simulink model "VelocityControl"  (R2018a)
settings: Solver=VariableStepAuto  StartTime=0.0  StopTime=10.0  RelTol=1e-3
values from neighbouring files (symbols this model uses):
  Dr = 30000    [BoatSim_config.m]    (also in WAM_V_config.mat)
  Du = 1000    [BoatSim_config.m]    (also in WAM_V_config.mat)
  Dv = 10000    [BoatSim_config.m]    (also in WAM_V_config.mat)
  IoM = ( 1 / 5 ) * Mass * ( ( Length / 2 )^2 + ( Width / 2 )^2 )    (= 4143.75)    [BoatSim_config.m]    (also in WAM_V_config.mat)
  Mass = 1500    [BoatSim_config.m]    (also in WAM_V_config.mat)
  rg = [ 0;0; ]    [BoatSim_config.m]    (also in WAM_V_config.mat = [0 0])
undefined symbols (not defined in the file or in its folder): X, Y, Z
libraries: robotlib x7, simulink x1
settings Model: Creator=ryodo  LastModifiedBy=ryodo

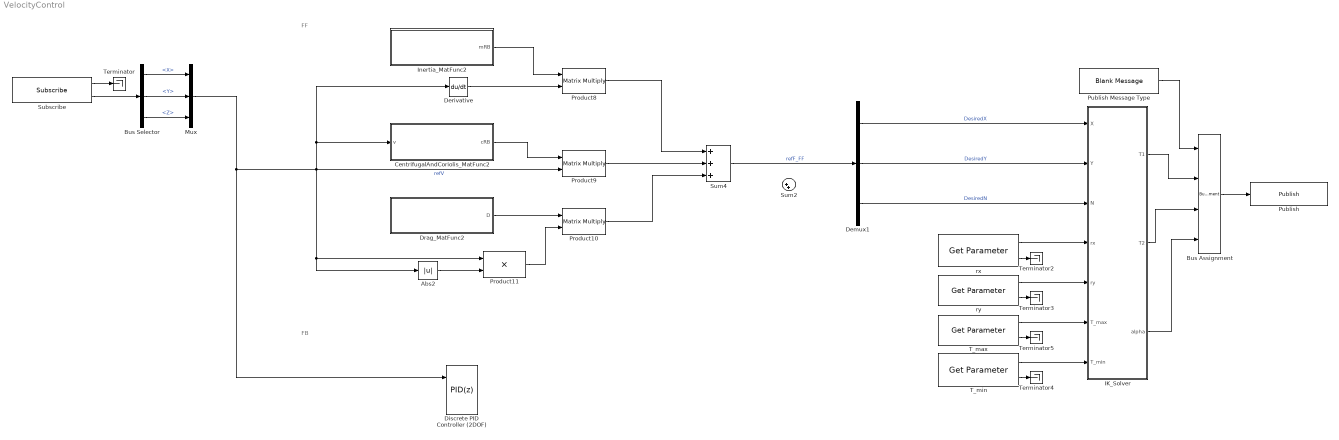
== system VelocityControl ==
  note: FF
  note: FB
  Abs2 : Abs
  Bus Assignment : BusAssignment  AssignedSignals=X,Y,Z
  Bus Selector : BusSelector  OutputSignals=Linear.X,Linear.Y,Angular.Z
  CentrifugalAndCoriolis_MatFunc2 : MATLAB Function  TreatAsAtomicUnit=on
  Demux1 : Demux  Outputs=3
  Derivative : Derivative
  Discrete PID Controller (2DOF) : simulink/Continuous/PID Controller (2DOF)  Controller=PID  TimeDomain=Discrete-time  SampleTime=-1  IntegratorMethod=Forward Euler  FilterMethod=Forward Euler  Form=Parallel  UseFilter=on  ControllerParametersSource=internal  P=1000  I=0  D=0  N=100  b=1  c=1  InitialConditionSource=internal  InitialConditionForIntegrator=0  InitialConditionForFilter=0  ExternalReset=none  ZeroCross=off  LimitOutput=off  UpperSaturationLimit=inf  LowerSaturationLimit=-inf  LinearizeAsGain=off  AntiWindupMode=none  Kb=1  TrackingMode=off  Kt=1  PParamMin=[]  PParamMax=[]  IParamMin=[]  IParamMax=[]  DParamMin=[]  DParamMax=[]  NParamMin=[]  NParamMax=[]  bParamMin=[]  bParamMax=[]  cParamMin=[]  cParamMax=[]  KbParamMin=[]  KbParamMax=[]  KtParamMin=[]  KtParamMax=[]  POutMin=[]  POutMax=[]  IOutMin=[]  IOutMax=[]  DOutMin=[]  DOutMax=[]  NOutMin=[]  NOutMax=[]  bOutMin=[]  bOutMax=[]  cOutMin=[]  cOutMax=[]  KbOutMin=[]  KbOutMax=[]  KtOutMin=[]  KtOutMax=[]  IntegratorOutMin=[]  IntegratorOutMax=[]  FilterOutMin=[]  FilterOutMax=[]  SumOutMin=[]  SumOutMax=[]  Sum1OutMin=[]  Sum1OutMax=[]  Sum2OutMin=[]  Sum2OutMax=[]  Sum3OutMin=[]  Sum3OutMax=[]  SumI1OutMin=[]  SumI1OutMax=[]  SumI2OutMin=[]  SumI2OutMax=[]  SumI3OutMin=[]  SumI3OutMax=[]  SumDOutMin=[]  SumDOutMax=[]  SaturationOutMin=[]  SaturationOutMax=[]  IntegratorContinuousStateAttributes=''  IntegratorStateMustResolveToSignalObject=off  IntegratorRTWStateStorageClass=Auto  FilterContinuousStateAttributes=''  FilterStateMustResolveToSignalObject=off  FilterRTWStateStorageClass=Auto  DifferentiatorICPrevScaledInput=0  DifferentiatorOutMin=[]  DifferentiatorOutMax=[]  FilterDiffOutCoefMin=[]  FilterDiffOutCoefMax=[]  SumDenOutMin=[]  SumDenOutMax=[]  SumNumOutMin=[]  SumNumOutMax=[]  ReciprocalOutMin=[]  ReciprocalOutMax=[]  DivideOutMin=[]  DivideOutMax=[]  TunerSelectOption=Transfer Function Based (PID Tuner App)
  Drag_MatFunc2 : MATLAB Function  TreatAsAtomicUnit=on
  IK_Solver : MATLAB Function  TreatAsAtomicUnit=on
  Inertia_MatFunc2 : MATLAB Function  TreatAsAtomicUnit=on
  Mux : Mux  Inputs=3
  Product10 : Product  Multiplication=Matrix(*)
  Product11 : Product
  Product8 : Product  Multiplication=Matrix(*)
  Product9 : Product  Multiplication=Matrix(*)
  Publish : robotlib/Publish  SourceLibraryInfo=This block requires Robotics System Toolbox  topicSource=Specify your own  topic=/result_force  messageType=geometry_msgs/Vector3  messageQueueLength=1
      settings: SourceProductBaseCode=RO
  Publish Message Type : robotlib/Blank Message  SourceLibraryInfo=This block requires Robotics System Toolbox  messageType=geometry_msgs/Vector3  SampleTime=-1
      settings: SourceProductBaseCode=RO
  Subscribe : robotlib/Subscribe  SourceLibraryInfo=This block requires Robotics System Toolbox  topicSource=Specify your own  topic=/cmd_vel  messageType=geometry_msgs/Twist  sampleTime=-1  messageQueueLength=1
      settings: SourceProductBaseCode=RO
  Sum2 : Sum  Inputs=|++
  Sum4 : Sum  Inputs=+++
  T_max : robotlib/Get Parameter  SourceLibraryInfo=This block requires Robotics System Toolbox  ParameterSource=Specify your own  ParameterName=/wam_v/T_max  ParameterType=double  ParameterMaxArrayLength=16  ParameterInitialValue=0.0  SampleTime=-1  ShowErrorCodeOutput=on  ModelName=VelocityControl  BlockId=ParamGet_VelocityControl_7
      settings: SourceProductName=Robotics System Toolbox  SourceProductBaseCode=RO
  T_min : robotlib/Get Parameter  SourceLibraryInfo=This block requires Robotics System Toolbox  ParameterSource=Specify your own  ParameterName=/wam_v/T_min  ParameterType=double  ParameterMaxArrayLength=16  ParameterInitialValue=0.0  SampleTime=-1  ShowErrorCodeOutput=on  ModelName=VelocityControl  BlockId=ParamGet_VelocityControl_8
      settings: SourceProductName=Robotics System Toolbox  SourceProductBaseCode=RO
  Terminator{,2..5} (5 alike) : Terminator
  rx : robotlib/Get Parameter  SourceLibraryInfo=This block requires Robotics System Toolbox  ParameterSource=Specify your own  ParameterName=/wam_v/rx  ParameterType=double  ParameterMaxArrayLength=16  ParameterInitialValue=0.0  SampleTime=-1  ShowErrorCodeOutput=on  ModelName=VelocityControl  BlockId=ParamGet_VelocityControl_14
      settings: SourceProductName=Robotics System Toolbox  SourceProductBaseCode=RO
  "ry " : robotlib/Get Parameter  SourceLibraryInfo=This block requires Robotics System Toolbox  ParameterSource=Specify your own  ParameterName=/wam_v/ry  ParameterType=double  ParameterMaxArrayLength=16  ParameterInitialValue=0.0  SampleTime=-1  ShowErrorCodeOutput=on  ModelName=VelocityControl  BlockId=ParamGet_VelocityControl_15
      settings: SourceProductName=Robotics System Toolbox  SourceProductBaseCode=RO
  wires:
  rx/2 -> Terminator2/1
  Bus Assignment/1 -> Publish/1
  T_min/2 -> Terminator4/1
  rx/1 -> IK_Solver/4(rx)
  IK_Solver/1(T1) -> Bus Assignment/2
  IK_Solver/3(alpha) -> Bus Assignment/4
  Publish Message Type/1 -> Bus Assignment/1
  T_min/1 -> IK_Solver/7(T_min)
  IK_Solver/2(T2) -> Bus Assignment/3
  "ry "/2 -> Terminator3/1
  T_max/1 -> IK_Solver/6(T_max)
  T_max/2 -> Terminator5/1
  "ry "/1 -> IK_Solver/5(ry)
  Drag_MatFunc2/1(D) -> Product10/1
  Bus Selector/2 -> Mux/2  "<Y>"
  Product8/1 -> Sum4/1
  Product9/1 -> Sum4/2
  Mux/1 -> Discrete PID Controller (2DOF)/1, Product11/1, Abs2/1, Derivative/1, CentrifugalAndCoriolis_MatFunc2/1(v), Product9/2  "refV"
  Product11/1 -> Product10/2
  Bus Selector/1 -> Mux/1  "<X>"
  Derivative/1 -> Product8/2
  CentrifugalAndCoriolis_MatFunc2/1(cRB) -> Product9/1
  Abs2/1 -> Product11/2
  Inertia_MatFunc2/1(mRB) -> Product8/1
  Bus Selector/3 -> Mux/3  "<Z>"
  Product10/1 -> Sum4/3
  Sum4/1 -> Demux1/1  "refF_FF"
  Subscribe/1 -> Terminator/1
  Demux1/1 -> IK_Solver/1(X)  "DesiredX"
  Demux1/2 -> IK_Solver/2(Y)  "DesiredY"
  Demux1/3 -> IK_Solver/3(N)  "DesiredN"
  Subscribe/2 -> Bus Selector/1

== matlab function VelocityControl/IK_Solver ==
  data: X input double size=1; T1 output double size=1; Y input double size=1; N input double size=1; T2 output double size=1; alpha output double size=1; rx input; ry input; T_max input; T_min input
function [ T1, T2, alpha ] = IK_Solver(X, Y, N, rx, ry, T_max, T_min)
    int8 x;
    int8 y;
    int8 n;
    x = 1 * int8(not(X==0));
    y = 2 * int8(not(Y==0));
    n = 4 * int8(not(N==0));

    switch x+y+n
        case 0
            T1=0;
            T2=0;
            alpha=0;
        case 1
            T1=X/2;
            T2=T1;
            alpha=0;
        case 2
            T1=Y/sqrt(2);
            T2=-T1;
            alpha=pi/4;
        case 3
            T1=(X+Y)/sqrt(2);
            T2=(X-Y)/sqrt(2);
            alpha=pi/4;
        case 4
            T1=N/(2*rx);
            T2=-T1;
            alpha=0;
        case 5
            T1=(X+(N/rx))/2;
            T2=(X-(N/rx))/2;
            alpha=0;
        case 6
            alpha=abs(atan((rx*Y)/(N+ry*Y)));
            double Ttmp_Y;
            double Ttmp_N;
            Ttmp_Y=Y/(2*sin(alpha));
            Ttmp_N=N/( 2*( rx*cos(alpha)-ry*sin(alpha) ) );
            if( (Ttmp_Y <= T_min || T_max <= Ttmp_Y) && (Ttmp_N <= T_min || T_max <= Ttmp_N) )
                T1=0;
                T2=0;
                alpha=0;
            elseif (Ttmp_Y <= T_min || T_max <= Ttmp_Y)
                T1=N/(2*rx);
                T2=-T1;
                alpha=0;
            elseif (Ttmp_N <= T_min || T_max <= Ttmp_N)
                T1=Y/sqrt(2);
                T2=-T1;
                alpha=pi/4;
            else
                T1=Ttmp_Y;
                T2=-T1;
            end
        case 7
            alpha=abs(atan((rx*Y)/(N+ry*Y)));
            double T1_tmp_Y;
            double T1_tmp_N;
            double T2_tmp_Y;
            double T2_tmp_N;
            T1_tmp_Y=X/(2*cos(alpha)) + Y/(2*sin(alpha));
            T1_tmp_N=X/(2*cos(alpha)) + N/( 2*(rx*cos(alpha)-ry*sin(alpha) ) );
            T2_tmp_Y=X/(2*cos(alpha)) - Y/(2*sin(alpha));    
            T2_tmp_N=X/(2*cos(alpha)) - N/( 2*(rx*cos(alpha)-ry*sin(alpha) ) );

            if( ( (T1_tmp_Y <= T_min || T_max <= T1_tmp_Y) || (T2_tmp_Y <= T_min || T_max <= T2_tmp_Y) ) && ( (T1_tmp_N <= T_min || T_max <= T1_tmp_N) || (T2_tmp_N <= T_min || T_max <= T2_tmp_N) ) )
                T1=0;
                T2=0;
                alpha=0;
            elseif ( (T1_tmp_Y <= T_min || T_max <= T1_tmp_Y) || (T2_tmp_Y <= T_min || T_max <= T2_tmp_Y) )
                T1=(X+(N/rx))/2;
                T2=(X-(N/rx))/2;
                alpha=0;
            elseif ( (T1_tmp_N <= T_min || T_max <= T1_tmp_N) || (T2_tmp_N <= T_min || T_max <= T2_tmp_N) )
                T1=(X+Y)/sqrt(2);
                T2=(X-Y)/sqrt(2);
                alpha=pi/4;
            else
                T1=T1_tmp_Y;
                T2=T2_tmp_Y;
            end
        otherwise
            T1=0;
            T2=0;
            alpha=0;
    end
    
%     Limit 
    if (T1 <= T_min)
        T1=T_min;
    end
    if (T_max <= T1)
        T1=T_max;
    end
    if (T2 <= T_min)
        T2=T_min;
    end
    if (T_max <= T2)
        T2=T_max;
    end
    if (alpha <= 0)
        alpha=0;
    end
    if (pi/2 <= alpha)
       alpha=pi/2;
    end

== matlab function VelocityControl/Inertia_MatFunc2 ==
  data: Mass parameter size=1; mRB output size=3,3; IoM parameter size=1; rg parameter size=2
function mRB = Inertia_MatFunc( Mass, IoM, rg )
    mRB = Inertia( Mass, IoM, rg );
end

== matlab function VelocityControl/CentrifugalAndCoriolis_MatFunc2 ==
  data: v input size=3; Mass parameter size=1; rg parameter size=2; cRB output size=3,3
function cRB = CentrifugalAndCoriolis_MatFunc( v, Mass, rg )
    cRB = CentrifugalAndCoriolis( Mass, rg, v );
end

== matlab function VelocityControl/Drag_MatFunc2 ==
  data: Du parameter size=1; Dv parameter size=1; D output size=3,3; Dr parameter size=1
function D = Drag_MatFunc( Du, Dv, Dr )
    D = Drag( Du, Dv, Dr );
end
